simulink model "sampleModel1809"  (R2023a)
settings: Solver=VariableStepAuto  StartTime=0.0  StopTime=10.0  RelTol=1e-3
libraries: hdlsllib x6, simulink x4
settings Model: Creator=user1  LastModifiedBy=user1

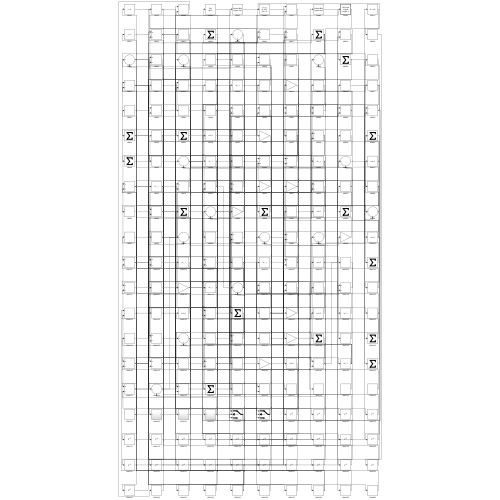
[thumbnail: Simulink's stored preview of the top-level diagram]
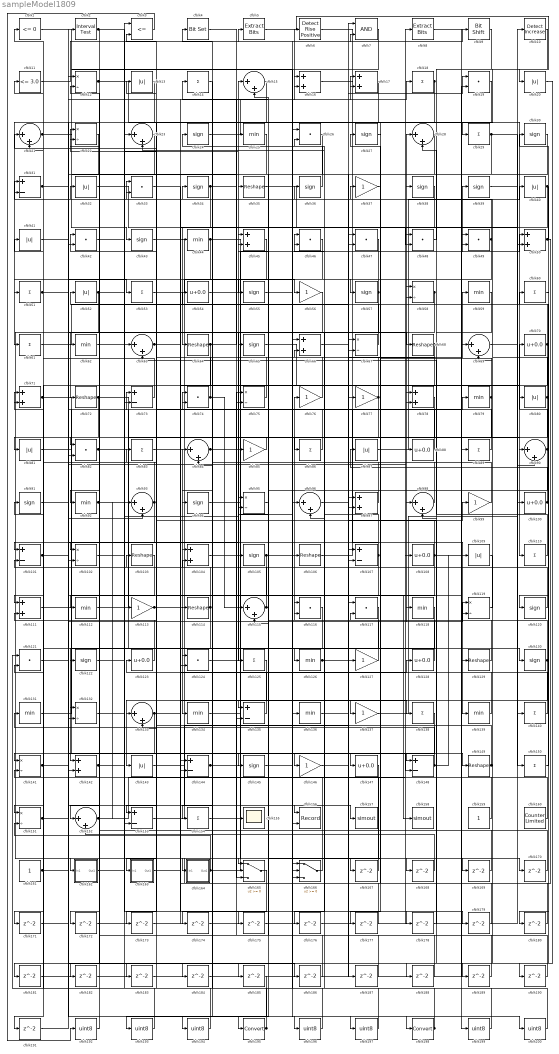
== system sampleModel1809 ==
  cfblk1 : hdlsllib/Logic and Bit Operations/Compare To Zero  relop=<=  OutDataTypeStr=boolean
  cfblk10 : simulink/Logic and Bit Operations/Detect Increase  vinit=0.0  OutDataTypeStr=boolean
      settings: LibrarySourceBlock=|
      | hdlsllib/Logic and Bit
      | Operations/Detect
      | Increase
  cfblk{54,70,88,100,108,123,128,147} (8 alike) : Bias  Bias=0.0  SaturateOnIntegerOverflow=off
  cfblk{31,73,101,107,135,144,148,153} (8 alike) : Sum  Inputs=+-
  cfblk{12,22,58,67,75,95,102,119,132,141,151} (11 alike) : Product  Inputs=*/  RndMeth=Zero  SaturateOnIntegerOverflow=on
  cfblk{35,64,68,72,103,106,114,129,149} (9 alike) : Reshape
  cfblk{16..17,45,50,66,71,78,97,104,111,142} (11 alike) : Sum
  cfblk{24,27,30,34,36,38..39,43,55,57,65,91,94,105,120,122,130,145} (18 alike) : Signum
  cfblk{13,20,32,40..41,52,80..81,87,109,143} (11 alike) : Abs  SaturateOnIntegerOverflow=off
  cfblk11 : hdlsllib/Logic and Bit Operations/Compare To Constant  relop=<=  const=3.0  OutDataTypeStr=boolean
  cfblk{14,18,29,51,53,60..61,83,86,89,110,125,138,140,150,154} (16 alike) : Sum  Inputs=+
  cfblk{25,44,59,62,79,92,112,118,126,131,134,136,139} (13 alike) : MinMax
  cfblk{37,56,76..77,85,99,113,127,137,146} (10 alike) : Gain
  cfblk{15,21,23,28,63,69,84,90,93,96,98,115,133,152} (14 alike) : Sum  Inputs=|++
  cfblk{19,26,33,42,46..49,74,82,116..117,121,124} (14 alike) : DotProduct  OutDataTypeStr=Inherit: Inherit via internal rule
  cfblk155 : Scope
  cfblk156 : Record  FileSettingsInternal="{\"entries\":[{\"content\":{\"excelSettings\":{\"content\":{},\"type\":\"Streamout.ExcelSettings\"}},\"type\":\"Streamout.FileSettingStorage\",\"uuid\":\"\"}],\"packageUris\":[\"http:\\/\\/schema.mathworks.com\\/mf0\\/streamout_blocks\\/R2020a\"],\"version\":\"1.0\"}"  Layout=[1 1]  SignalsInternal="{\"entries\":[{\"content\":{},\"type\":\"RecordBlkView.InputSignals\",\"uuid\":\"\"}],\"packageUris\":[\"http:\\/\\/schema.mathworks.com\\/mf0\\/streamout_blocks\\/R2020a\"],\"version\":\"1.0\"}"  VisualizationBindings="{\"xyplotplugin\":{\"info\":[{\"series\":[{\"bindingParametersList\":[{\"parameter\":\"X-Axis\",\"signalID\":4216,\"signalName\":\"cfblk122\"},{\"parameter\":\"Y-Axis\",\"signalID\":4220,\"signalName\":\"cfblk101\"}],\"seriesID\":39729}],\"subplotID\":1}]}}"  CompatibilityTag=XY  st=-1
  cfblk157 : ToWorkspace  VariableName=simout  SaveFormat=Timeseries  SampleTime=-1
  cfblk158 : ToWorkspace  VariableName=simout  SaveFormat=Timeseries  SampleTime=-1
  cfblk159 : Constant  SampleTime=-1
  cfblk160 : hdlsllib/Sources/Counter Limited  uplimit=7  tsamp=-1
  cfblk161 : Constant  SampleTime=-1
  cfblk162 : Subsystem
      settings: LibrarySourceBlock=|
      | hdlsllib/Ports &
      | Subsystems/Subsystem
  cfblk163 : Subsystem
      settings: LibrarySourceBlock=|
      | hdlsllib/Ports &
      | Subsystems/Subsystem
  cfblk164 : Subsystem
      settings: LibrarySourceBlock=|
      | hdlsllib/Ports &
      | Subsystems/Subsystem
  cfblk165 : Switch  SaturateOnIntegerOverflow=off  InputSameDT=off
  cfblk166 : Switch  SaturateOnIntegerOverflow=off  InputSameDT=off
  cfblk{167..191} (25 alike) : Delay  SampleTime=1
  cfblk{192..194,196..197,199..200} (7 alike) : DataTypeConversion  OutDataTypeStr=uint8  SaturateOnIntegerOverflow=off  RndMeth=Floor
  cfblk195 : DataTypeConversion  SaturateOnIntegerOverflow=off  RndMeth=Floor
  cfblk198 : DataTypeConversion  SaturateOnIntegerOverflow=off  RndMeth=Floor
  cfblk2 : hdlsllib/Logic and Bit Operations/Interval Test  IntervalClosedRight=on  uplimit=0.5  IntervalClosedLeft=on  lowlimit=-0.5  OutDataTypeStr=boolean
  cfblk3 : RelationalOperator  Operator=<=  OutDataTypeStr=boolean  InputSameDT=off
  cfblk4 : simulink/Logic and Bit Operations/Bit Set  iBit=0
      settings: LibrarySourceBlock=|
      | hdlsllib/Logic and Bit
      | Operations/Bit Set
  cfblk5 : simulink/Logic and Bit Operations/Extract Bits  bitsToExtract=Upper half  numBits=8  bitIdxRange=[0 7]  outScalingMode=Preserve fixed-point scaling
      settings: LibrarySourceBlock=|
      | hdlsllib/Logic and Bit
      | Operations/Extract Bits
  cfblk6 : hdlsllib/Logic and Bit Operations/Detect Rise Positive  vinit=0  OutDataTypeStr=boolean
  cfblk7 : Logic  AllPortsSameDT=off  OutDataTypeStr=boolean
  cfblk8 : simulink/Logic and Bit Operations/Extract Bits  bitsToExtract=Upper half  numBits=8  bitIdxRange=[0 7]  outScalingMode=Preserve fixed-point scaling
      settings: LibrarySourceBlock=|
      | hdlsllib/Logic and Bit
      | Operations/Extract Bits
  cfblk9 : hdlsllib/Logic and Bit Operations/Bit Shift  mode=Shift Left Logical  N=0
  wires:
  cfblk111/1 -> cfblk126/1
  cfblk128/1 -> cfblk28/1
  cfblk12/1 -> cfblk110/1, cfblk7/2, cfblk82/1
  cfblk71/1 -> cfblk158/1, cfblk93/2
  cfblk7/1 -> cfblk43/1
  cfblk72/1 -> cfblk130/1, cfblk132/2
  cfblk52/1 -> cfblk162/1(In1), cfblk25/1
  cfblk131/1 -> cfblk73/1
  cfblk106/1 -> cfblk79/1
  cfblk81/1 -> cfblk146/1
  cfblk86/1 -> cfblk42/1
  cfblk80/1 -> cfblk38/1, cfblk144/2, cfblk145/1
  cfblk150/1 -> cfblk60/1
  cfblk113/1 -> cfblk137/1, cfblk16/2
  cfblk43/1 -> cfblk157/1
  cfblk125/1 -> cfblk143/1
  cfblk117/1 -> cfblk142/1
  cfblk105/1 -> cfblk166/1, cfblk173/1
  cfblk40/1 -> cfblk64/1, cfblk190/1
  cfblk119/1 -> cfblk59/1
  cfblk134/1 -> cfblk50/1
  cfblk53/1 -> cfblk56/1
  cfblk67/1 -> cfblk15/1
  cfblk136/1 -> cfblk107/1
  cfblk11/1 -> cfblk5/1
  cfblk151/1 -> cfblk78/1, cfblk196/1
  cfblk48/1 -> cfblk28/2
  cfblk85/1 -> cfblk81/1
  cfblk87/1 -> cfblk40/1
  cfblk54/1 -> cfblk149/1
  cfblk112/1 -> cfblk58/1
  cfblk6/1 -> cfblk139/1
  cfblk13/1 -> cfblk61/1
  cfblk38/1 -> cfblk48/2
  cfblk36/1 -> cfblk24/1
  cfblk83/1 -> cfblk134/1
  cfblk120/1 -> cfblk71/1
  cfblk2/1 -> cfblk102/1, cfblk164/1(In1)
  cfblk126/1 -> cfblk77/1, cfblk69/1, cfblk99/1
  cfblk137/1 -> cfblk10/1
  cfblk27/1 -> cfblk147/1
  cfblk143/1 -> cfblk127/1
  cfblk152/1 -> cfblk8/1, cfblk93/1
  cfblk127/1 -> cfblk76/1
  cfblk39/1 -> cfblk100/1
  cfblk9/1 -> cfblk98/2
  cfblk148/1 -> cfblk131/1, cfblk109/1
  cfblk98/1 -> cfblk46/1
  cfblk96/1 -> cfblk117/1
  cfblk14/1 -> cfblk124/1
  cfblk164/1(Out1) -> cfblk118/1, cfblk151/2
  cfblk35/1 -> cfblk129/1
  cfblk64/1 -> cfblk152/1, cfblk18/1
  cfblk31/1 -> cfblk53/1, cfblk166/3, cfblk68/1
  cfblk99/1 -> cfblk58/2
  cfblk94/1 -> cfblk166/2
  cfblk5/1 -> cfblk20/1
  cfblk124/1 -> cfblk45/1
  cfblk153/1 -> cfblk96/1
  cfblk22/1 -> cfblk42/2
  cfblk44/1 -> cfblk90/1, cfblk153/2
  cfblk55/1 -> cfblk9/1
  cfblk82/1 -> cfblk86/1, cfblk119/2
  cfblk57/1 -> cfblk125/1, cfblk62/1, cfblk55/1, cfblk135/2
  cfblk154/1 -> cfblk106/1
  cfblk16/1 -> cfblk90/2
  cfblk51/1 -> cfblk12/1, cfblk148/1
  cfblk74/1 -> cfblk52/1, cfblk115/1
  cfblk50/1 -> cfblk165/1, cfblk30/1
  cfblk135/1 -> cfblk123/1
  cfblk41/1 -> cfblk17/1
  cfblk90/1 -> cfblk70/1, cfblk115/2
  cfblk25/1 -> cfblk94/1
  cfblk15/1 -> cfblk154/1
  cfblk100/1 -> cfblk87/1, cfblk69/2, cfblk120/1
  cfblk102/1 -> cfblk23/1
  cfblk166/1 -> cfblk95/1
  cfblk76/1 -> cfblk21/1
  cfblk103/1 -> cfblk142/2
  cfblk115/1 -> cfblk22/1, cfblk135/1, cfblk71/2
  cfblk146/1 -> cfblk19/1
  cfblk26/1 -> cfblk195/1
  cfblk68/1 -> cfblk114/1, cfblk66/2
  cfblk46/1 -> cfblk51/1
  cfblk114/1 -> cfblk33/1, cfblk133/2
  cfblk61/1 -> cfblk7/1
  cfblk21/1 -> cfblk155/1, cfblk169/1
  cfblk159/1 -> cfblk103/1
  cfblk56/1 -> cfblk133/1
  cfblk70/1 -> cfblk13/1, cfblk111/1
  cfblk141/1 -> cfblk88/1, cfblk184/1, cfblk186/1
  cfblk160/1 -> cfblk116/1
  cfblk1/1 -> cfblk136/1
  cfblk144/1 -> cfblk108/1, cfblk78/2
  cfblk49/1 -> cfblk67/2, cfblk31/2
  cfblk32/1 -> cfblk97/1
  cfblk47/1 -> cfblk57/1
  cfblk89/1 -> cfblk34/1
  cfblk18/1 -> cfblk44/1, cfblk73/2, cfblk82/2
  cfblk78/1 -> cfblk141/1
  cfblk28/1 -> cfblk102/2
  cfblk162/1(Out1) -> cfblk113/1
  cfblk161/1 -> cfblk21/2, cfblk119/1
  cfblk65/1 -> cfblk89/1
  cfblk108/1 -> cfblk19/2, cfblk33/2, cfblk153/1
  cfblk139/1 -> cfblk27/1
  cfblk142/1 -> cfblk95/2, cfblk16/1
  cfblk23/1 -> cfblk112/1
  cfblk92/1 -> cfblk66/1, cfblk85/1
  cfblk34/1 -> cfblk124/2, cfblk80/1
  cfblk42/1 -> cfblk17/2
  cfblk63/1 -> cfblk138/1, cfblk105/1, cfblk75/2
  cfblk130/1 -> cfblk14/1, cfblk174/1
  cfblk10/1 -> cfblk29/1
  cfblk29/1 -> cfblk140/1, cfblk47/2
  cfblk30/1 -> cfblk92/1
  cfblk97/1 -> cfblk74/1
  cfblk129/1 -> cfblk36/1
  cfblk123/1 -> cfblk11/1
  cfblk73/1 -> cfblk41/1
  cfblk84/1 -> cfblk39/1, cfblk148/2
  cfblk17/1 -> cfblk163/1(In1)
  cfblk110/1 -> cfblk63/2
  cfblk88/1 -> cfblk35/1
  cfblk24/1 -> cfblk6/1
  cfblk149/1 -> cfblk116/2, cfblk96/2, cfblk111/2
  cfblk121/1 -> cfblk198/1
  cfblk93/1 -> cfblk31/1, cfblk182/1
  cfblk79/1 -> cfblk37/1, cfblk84/2
  cfblk104/1 -> cfblk49/2
  cfblk122/1 -> cfblk156/1
  cfblk101/1 -> cfblk104/1, cfblk156/2
  cfblk140/1 -> cfblk4/1
  cfblk107/1 -> cfblk101/1, cfblk23/2, cfblk165/3
  cfblk75/1 -> cfblk65/1
  cfblk95/1 -> cfblk45/2
  cfblk69/1 -> cfblk150/1
  cfblk133/1 -> cfblk128/1, cfblk151/1
  cfblk58/1 -> cfblk72/1, cfblk176/1
  cfblk116/1 -> cfblk132/1
  cfblk77/1 -> cfblk122/1, cfblk22/2
  cfblk37/1 -> cfblk167/1
  cfblk167/1 -> cfblk1/1
  cfblk4/1 -> cfblk168/1
  cfblk168/1 -> cfblk152/2
  cfblk169/1 -> cfblk74/2
  cfblk62/1 -> cfblk170/1
  cfblk170/1 -> cfblk101/2
  cfblk138/1 -> cfblk171/1
  cfblk45/1 -> cfblk172/1
  cfblk172/1 -> cfblk97/2
  cfblk173/1 -> cfblk84/1
  cfblk174/1 -> cfblk107/2
  cfblk132/1 -> cfblk175/1
  cfblk175/1 -> cfblk48/1
  cfblk176/1 -> cfblk50/2
  cfblk19/1 -> cfblk177/1
  cfblk177/1 -> cfblk144/1
  cfblk33/1 -> cfblk178/1
  cfblk178/1 -> cfblk98/1
  cfblk163/1(Out1) -> cfblk179/1
  cfblk179/1 -> cfblk75/1
  cfblk60/1 -> cfblk180/1
  cfblk180/1 -> cfblk117/2
  cfblk20/1 -> cfblk181/1
  cfblk181/1 -> cfblk63/1
  cfblk182/1 -> cfblk49/1
  cfblk91/1 -> cfblk183/1
  cfblk183/1 -> cfblk47/1
  cfblk184/1 -> cfblk67/1
  cfblk147/1 -> cfblk185/1
  cfblk186/1 -> cfblk165/2
  cfblk66/1 -> cfblk187/1
  cfblk187/1 -> cfblk15/2
  cfblk59/1 -> cfblk188/1
  cfblk188/1 -> cfblk12/2
  cfblk109/1 -> cfblk189/1
  cfblk189/1 -> cfblk46/2
  cfblk190/1 -> cfblk104/2
  cfblk118/1 -> cfblk191/1
  cfblk191/1 -> cfblk2/1
  cfblk3/1 -> cfblk192/1
  cfblk192/1 -> cfblk32/1
  cfblk185/1 -> cfblk193/1
  cfblk193/1 -> cfblk3/1
  cfblk165/1 -> cfblk194/1
  cfblk194/1 -> cfblk3/2
  cfblk195/1 -> cfblk141/2, cfblk91/1
  cfblk196/1 -> cfblk26/1
  cfblk145/1 -> cfblk197/1
  cfblk197/1 -> cfblk26/2
  cfblk198/1 -> cfblk54/1, cfblk83/1
  cfblk8/1 -> cfblk199/1
  cfblk199/1 -> cfblk121/1
  cfblk171/1 -> cfblk200/1
  cfblk200/1 -> cfblk121/2

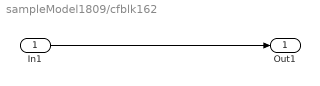
== system sampleModel1809/cfblk162 ==
  In1 : Inport
  Out1 : Outport
  wires:
  In1/1 -> Out1/1

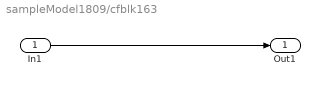
== system sampleModel1809/cfblk163 ==
  In1 : Inport
  Out1 : Outport
  wires:
  In1/1 -> Out1/1

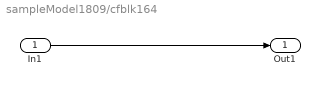
== system sampleModel1809/cfblk164 ==
  In1 : Inport
  Out1 : Outport
  wires:
  In1/1 -> Out1/1
